simulink model "LQG_AWBT"  (R2015a)
settings: Solver=ode5  StartTime=0.0  StopTime=10  FixedStep=1e-4  RelTol=1e-3
values from neighbouring files (symbols this model uses):
  Ak = inv(P12)*(A_hat-P12*Bk*Cy*Q11-P11*Bp*Ck*Q12'-P11*(Ap+Bp*Dk*Cy)*Q11)*inv(Q12')    [finding_Q12P12.m]    (also in main_matlab_LMI_Theorem4.m; main_matlab_LMI_Theorem5.m)
  Bk = inv(P12)*(B_hat-P11*Bp*Dk)    [finding_Q12P12.m]    (also in main_matlab_LMI_Theorem4.m; main_matlab_LMI_Theorem5.m)
  Ck = (C_hat-Dk*Cy*Q11)*inv(Q12')    [finding_Q12P12.m]    (also in main_matlab_LMI_Theorem4.m; main_matlab_LMI_Theorem5.m)
  Dk = D_hat    [finding_Q12P12.m]    (also in main_matlab_LMI_Theorem4.m; main_matlab_LMI_Theorem5.m)
  Lambda = [GAMA1;GAMA2]    [main_matlab_LMI_Theorem4.m]
  nk = sqrt(numel(Ak))    [main_matlab_LMI_Theorem4.m]    (also in main_matlab_LMI_Theorem5.m)
  nu = numel(Bp)/np    [main_matlab_LMI_Theorem4.m]    (also in main_matlab_LMI_Theorem5.m)
undefined symbols (not defined in the file or in its folder): Af, Bf, Cf, Hf
settings Model: Creator=p4wp4w  LastModifiedBy=Ablah

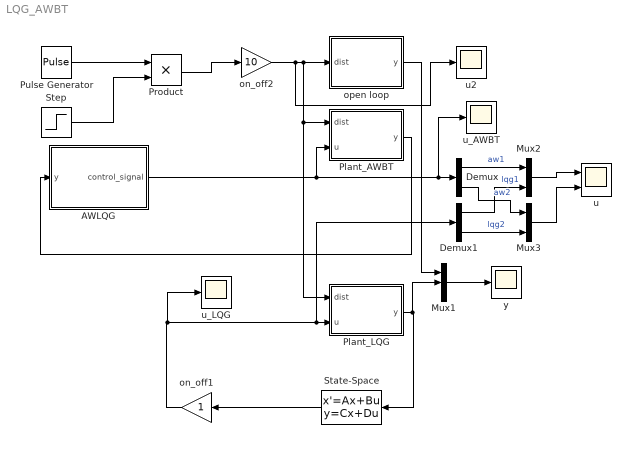
== system LQG_AWBT ==
  AWLQG : Subsystem
  Demux : Demux  Outputs=2
  Demux1 : Demux  Outputs=2
  Mux1 : Mux  Inputs=3
  Mux2 : Mux  Inputs=2
  Mux3 : Mux  Inputs=2
  Plant_AWBT : Subsystem
  Plant_LQG : Subsystem
  Product : Product
  Pulse Generator : DiscretePulseGenerator  PulseType=Time based  Period=0.5  PulseWidth=10
  State-Space : StateSpace  A=Ak  B=Bk  C=Ck  D=Dk  X0=0
  Step : Step  Time=0.5  Before=1  After=0  SampleTime=0
  on_off1 : Gain
  on_off2 : Gain  Gain=10
  open loop : Subsystem
  u : Scope  NumInputPorts=2
      settings: ShowLegends=on  YMin=-7.5~-5  YMax=7.5~4  SaveName=ScopeData3
  u2 : Scope
      settings: ShowLegends=on  YMin=-0.8  YMax=0.7  SaveName=ScopeData6
  u_AWBT : Scope
      settings: YMin=-1  YMax=1
  u_LQG : Scope
      settings: SaveName=ScopeData2
  y : Scope
      settings: ShowLegends=on  YMin=-15  YMax=15
  wires:
  State-Space/1 -> on_off1/1
  Mux1/1 -> y/1
  open loop/1(y) -> Mux1/1
  on_off1/1 -> u_LQG/1, Demux1/1, Plant_LQG/2(u)
  on_off2/1 -> u2/1, open loop/1(dist), Plant_LQG/1(dist), Plant_AWBT/1(dist)
  Plant_LQG/1(y) -> State-Space/1, Mux1/2
  Plant_AWBT/1(y) -> AWLQG/1(y)
  Demux/1 -> Mux2/1  "aw1"
  Demux1/1 -> Mux2/2  "lqg1"
  Demux/2 -> Mux3/1  "aw2"
  Demux1/2 -> Mux3/2  "lqg2"
  Mux2/1 -> u/1
  Mux3/1 -> u/2
  AWLQG/1(control_signal) -> Plant_AWBT/2(u), u_AWBT/1, Demux/1
  Pulse Generator/1 -> Product/1
  Step/1 -> Product/2
  Product/1 -> on_off2/1

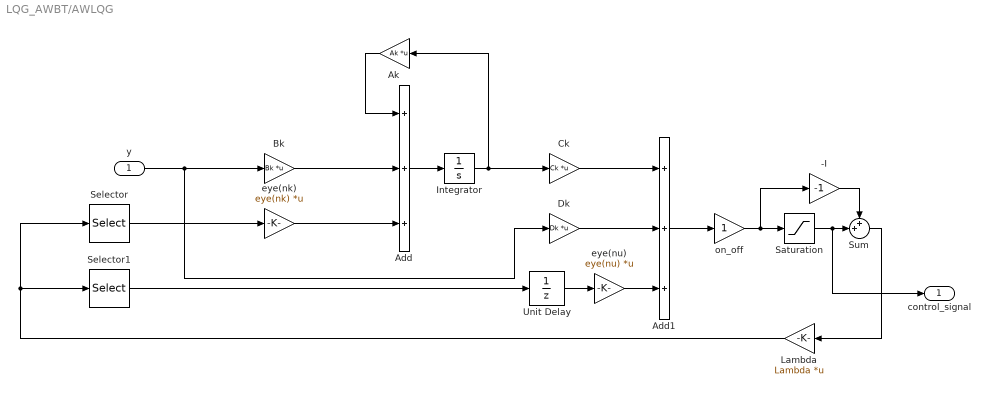
== system LQG_AWBT/AWLQG ==
  y : Inport
  -I : Gain  Gain=-1
  Add : Sum  Inputs=+++
  Add1 : Sum  Inputs=+++
  Ak : Gain  Gain=Ak  Multiplication=Matrix(K*u)
  Bk : Gain  Gain=Bk  Multiplication=Matrix(K*u)
  Ck : Gain  Gain=Ck  Multiplication=Matrix(K*u)
  Dk : Gain  Gain=Dk  Multiplication=Matrix(K*u)
  Integrator : Integrator
  Lambda : Gain  Gain=Lambda  Multiplication=Matrix(K*u)
  Saturation : Saturate  UpperLimit=2  LowerLimit=-2
  Selector : Selector  InputPortWidth=nk+nu  Indices=[1:nk]
  Selector1 : Selector  InputPortWidth=nk+nu  Indices=[nk+1:nk+nu]
  Sum : Sum  Inputs=++|
  Unit Delay : UnitDelay  SampleTime=-1
  eye(nk) : Gain  Gain=eye(nk)  Multiplication=Matrix(K*u)
  eye(nu) : Gain  Gain=eye(nu)  Multiplication=Matrix(K*u)
  on_off : Gain
  control_signal : Outport
  wires:
  Lambda/1 -> Selector1/1, Selector/1
  -I/1 -> Sum/1
  Sum/1 -> Lambda/1
  Add1/1 -> on_off/1
  Saturation/1 -> control_signal/1, Sum/2
  on_off/1 -> -I/1, Saturation/1
  Add/1 -> Integrator/1
  Integrator/1 -> Ak/1, Ck/1
  Ak/1 -> Add/1
  Bk/1 -> Add/2
  y/1 -> Dk/1, Bk/1
  eye(nk)/1 -> Add/3
  Selector/1 -> eye(nk)/1
  Ck/1 -> Add1/1
  Dk/1 -> Add1/2
  eye(nu)/1 -> Add1/3
  Selector1/1 -> Unit Delay/1
  Unit Delay/1 -> eye(nu)/1

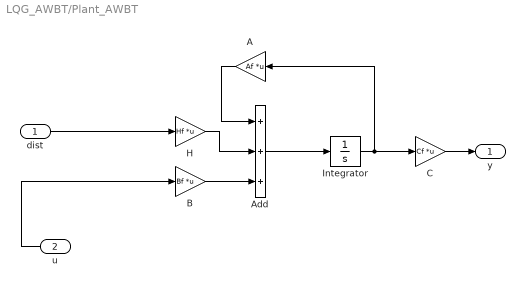
== system LQG_AWBT/Plant_AWBT ==
  dist : Inport
  u : Inport  Port=2
  A : Gain  Gain=Af  Multiplication=Matrix(K*u)
  Add : Sum  Inputs=+++
  B : Gain  Gain=Bf  Multiplication=Matrix(K*u)
  C : Gain  Gain=Cf  Multiplication=Matrix(K*u)
  H : Gain  Gain=Hf  Multiplication=Matrix(K*u)
  Integrator : Integrator
  y : Outport
  wires:
  Add/1 -> Integrator/1
  H/1 -> Add/2
  A/1 -> Add/1
  dist/1 -> H/1
  C/1 -> y/1
  B/1 -> Add/3
  Integrator/1 -> C/1, A/1
  u/1 -> B/1

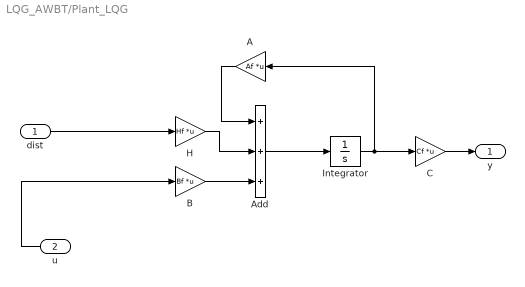
== system LQG_AWBT/Plant_LQG ==
  dist : Inport
  u : Inport  Port=2
  A : Gain  Gain=Af  Multiplication=Matrix(K*u)
  Add : Sum  Inputs=+++
  B : Gain  Gain=Bf  Multiplication=Matrix(K*u)
  C : Gain  Gain=Cf  Multiplication=Matrix(K*u)
  H : Gain  Gain=Hf  Multiplication=Matrix(K*u)
  Integrator : Integrator
  y : Outport
  wires:
  u/1 -> B/1
  Integrator/1 -> A/1, C/1
  B/1 -> Add/3
  C/1 -> y/1
  dist/1 -> H/1
  A/1 -> Add/1
  H/1 -> Add/2
  Add/1 -> Integrator/1

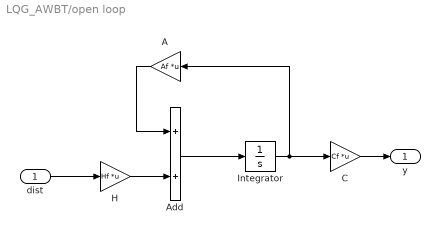
== system LQG_AWBT/open loop ==
  dist : Inport
  A : Gain  Gain=Af  Multiplication=Matrix(K*u)
  Add : Sum
  C : Gain  Gain=Cf  Multiplication=Matrix(K*u)
  H : Gain  Gain=Hf  Multiplication=Matrix(K*u)
  Integrator : Integrator
  y : Outport
  wires:
  Integrator/1 -> A/1, C/1
  C/1 -> y/1
  dist/1 -> H/1
  A/1 -> Add/1
  H/1 -> Add/2
  Add/1 -> Integrator/1
